simulink model "MMC_AverageModel_20250509"  (R2024b)
settings: Solver=VariableStepAuto  StartTime=0.0  StopTime=0.5  RelTol=1e-3
values from neighbouring files (symbols this model uses):
  Ceq = 3e-3    (= 0.003)    [param_allsim_20250429.m]
  f0 = 50    [param_allsim_20250429.m]
  L_ac = 100e-6    (= 0.0001)    [param_allsim_20250429.m]
  L_arm = 1e-3    (= 0.001)    [param_allsim_20250429.m]
  m_Delta_d = M_Delta*sin(Phi_Delta)    [param_allsim_20250429.m]
  m_Delta_q = -M_Delta*cos(Phi_Delta)    [param_allsim_20250429.m]
  m_Sigma_0 = m_Sigma_0_n    (= 1)    [param_allsim_20250429.m]
  m_Sigma_d = M_Sigma*sin(Phi_Sigma)    [param_allsim_20250429.m]
  m_Sigma_q = -M_Sigma*cos(Phi_Sigma)    [param_allsim_20250429.m]
  R_ac = 1    [param_allsim_20250429.m]
  R_arm = 1e-2    (= 0.01)    [param_allsim_20250429.m]
  VDC = 800    [param_allsim_20250429.m]
undefined symbols (not defined in the file or in its folder): C_SM, Rc
libraries: spsVoltageMeasurementLib x12, spsSeriesRLCBranchLib x12, spsCurrentMeasurementLib x10, spsControlledCurrentSourceLib x6, spsControlledVoltageSourceLib x6, spsabctodq0Lib x6, spsDCVoltageSourceLib x2, spsMeanLib x2, spsdq0toabcLib x2, spsGroundLib x1, spsThreePhaseSeriesRLCBranchLib x1, spspowerguiLib x1
settings Model: Creator=ana  LastModifiedBy=ana

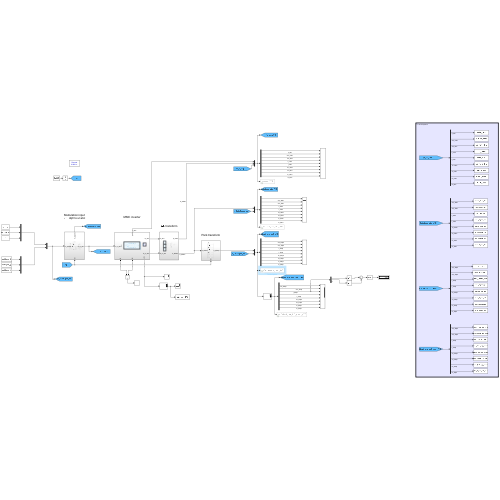
[thumbnail: Simulink's stored preview of the top-level diagram]
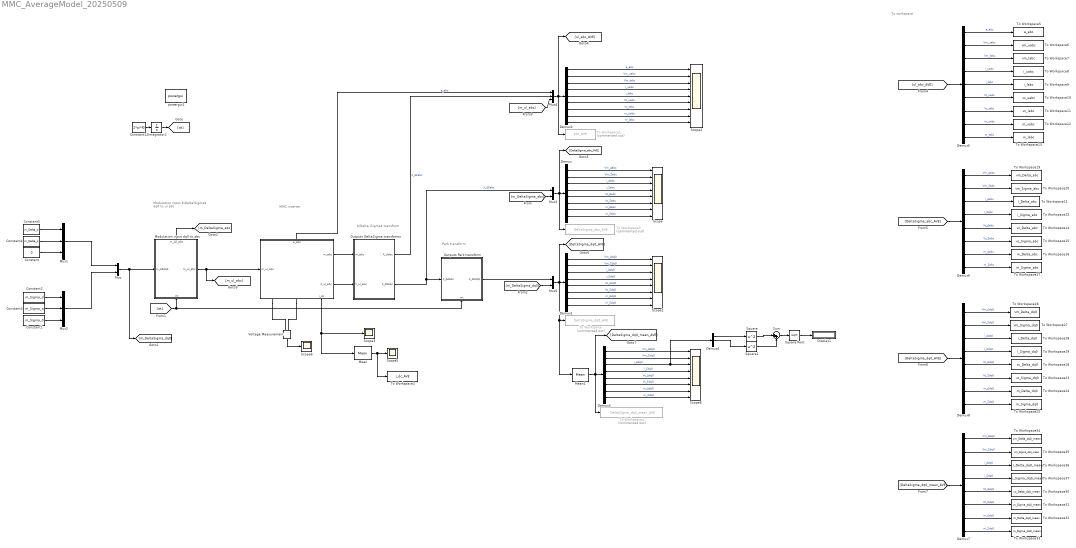
== system MMC_AverageModel_20250509 ==
  note: MMC inverter
  note: $\Delta \Sigma$ transform
  note: Modulation input
      | $\Delta\Sigma$ dq0 to ul abc
  note: Park transform
  note: To workspace
  " " : Subsystem
      settings: PortSchema="{\"entries\":[{\"content\":{\"sides\":[{\"content\":{\"connectorIds\":[\"In1\"]},\"type\":\"ConnectorPlacement.EquallySpacedRectSide\",\"uuid\":\"be96b836-162a-4026-8928-e777e4800056\"},{\"content\":{\"connectorIds\":[\"Out1\",\"Out2\"],\"side\":\"RIGHT\"},\"type\":\"ConnectorPlacement.EquallySpacedRectSide\",\"uuid\":\"77a090ea-e307-4fed-ac75-684872a04d06\"},{\"content\":{\"connectorIds\":[\"Out4\"],\"side\":\"TOP\"},\"type\":\"ConnectorPlacement.EquallySpacedRectSide\",\"uuid\":\"73b87893-2e5b-4437-8911-e3d659e39832\"},{\"content\":{\"connectorIds\":[\"RConn1\",\"RConn2\",\"Out3\"],\"side\":\"BOTTOM\"},\"type\":\"ConnectorPlacement.EquallySpacedRectSide\",\"uuid\":\"828178e9-16e3-463b-9057-d6fa245d9764\"}]},\"type\":\"ConnectorPlacement.EquallySpacedConnector\",\"uuid\":\"6b316bfb-7390-469c-962b-5ea2d8aa7073\"}],\"packageUris\":[\"http://schema.mathworks.com/mf0/Connector/R2020b\"],\"version\":\"1.0\"}"
  Constant : Constant  Value=0
  Constant1 : Constant  Value=m_Sigma_0
  Constant12 : Constant  Value=2*pi*f0
  Constant2 : Constant  Value=m_Sigma_d
  Constant3 : Constant  Value=m_Sigma_q
  Constant4 : Constant  Value=m_Delta_q
  Constant5 : Constant  Value=m_Delta_d
  Demux{,1,3,6..8} (6 alike) : Demux  Outputs=8
  Demux2 : Demux  Outputs=9
  Demux4 : Demux  Outputs=3
  Demux5 : Demux  Outputs=9
  Display1 : Display
  Integrator2 : Integrator
  Mean : spsMeanLib/Mean  Freq=500  Vinit=0  Ts=0
  Mean1 : spsMeanLib/Mean  Freq=500  Vinit=0  Ts=0
  Modulation input dq0 to abc : Subsystem
      settings: PortSchema="{\"entries\":[{\"content\":{\"sides\":[{\"content\":{\"connectorIds\":[\"Out2\"]},\"type\":\"ConnectorPlacement.EquallySpacedRectSide\",\"uuid\":\"c93fa5b4-0f06-4bab-a3ea-c283951bfaa2\"},{\"content\":{\"connectorIds\":[\"In2\"],\"side\":\"RIGHT\"},\"type\":\"ConnectorPlacement.EquallySpacedRectSide\",\"uuid\":\"754fc415-ee26-4c64-88d9-9fe4c190d1ce\"},{\"content\":{\"connectorIds\":[\"Out1\"],\"side\":\"TOP\"},\"type\":\"ConnectorPlacement.EquallySpacedRectSide\",\"uuid\":\"5a2ac060-a673-4c08-b077-b80c57d082e2\"},{\"content\":{\"connectorIds\":[\"In1\"],\"side\":\"BOTTOM\"},\"type\":\"ConnectorPlacement.EquallySpacedRectSide\",\"uuid\":\"ce66d6e2-1782-404f-a52c-1b3df510631d\"}]},\"type\":\"ConnectorPlacement.EquallySpacedConnector\",\"uuid\":\"907f6fc0-1e89-4b6d-bca9-d0cf84d5397d\"}],\"packageUris\":[\"http://schema.mathworks.com/mf0/Connector/R2020b\"],\"version\":\"1.0\"}"
  Mux : Mux  Inputs=2
  Mux1 : Mux  Inputs=3
  Mux2 : Mux  Inputs=3
  Mux3 : Mux  Inputs=2
  Mux4 : Mux  Inputs=3
  Mux5 : Mux  Inputs=2
  Outputs DeltaSigma transforms : Subsystem
      settings: PortSchema="{\"entries\":[{\"content\":{\"sides\":[{\"content\":{\"connectorIds\":[\"Out1\",\"Out2\"]},\"type\":\"ConnectorPlacement.EquallySpacedRectSide\",\"uuid\":\"c93fa5b4-0f06-4bab-a3ea-c283951bfaa2\"},{\"content\":{\"connectorIds\":[\"In1\",\"In2\"],\"side\":\"RIGHT\"},\"type\":\"ConnectorPlacement.EquallySpacedRectSide\",\"uuid\":\"754fc415-ee26-4c64-88d9-9fe4c190d1ce\"},{\"content\":{\"side\":\"TOP\"},\"type\":\"ConnectorPlacement.EquallySpacedRectSide\",\"uuid\":\"5a2ac060-a673-4c08-b077-b80c57d082e2\"},{\"content\":{\"side\":\"BOTTOM\"},\"type\":\"ConnectorPlacement.EquallySpacedRectSide\",\"uuid\":\"ce66d6e2-1782-404f-a52c-1b3df510631d\"}]},\"type\":\"ConnectorPlacement.EquallySpacedConnector\",\"uuid\":\"907f6fc0-1e89-4b6d-bca9-d0cf84d5397d\"}],\"packageUris\":[\"http://schema.mathworks.com/mf0/Connector/R2020b\"],\"version\":\"1.0\"}"
  Outputs Park transform : Subsystem
      settings: PortSchema="{\"entries\":[{\"content\":{\"sides\":[{\"content\":{\"connectorIds\":[\"Out1\"]},\"type\":\"ConnectorPlacement.EquallySpacedRectSide\",\"uuid\":\"c93fa5b4-0f06-4bab-a3ea-c283951bfaa2\"},{\"content\":{\"connectorIds\":[\"In2\"],\"side\":\"RIGHT\"},\"type\":\"ConnectorPlacement.EquallySpacedRectSide\",\"uuid\":\"754fc415-ee26-4c64-88d9-9fe4c190d1ce\"},{\"content\":{\"side\":\"TOP\"},\"type\":\"ConnectorPlacement.EquallySpacedRectSide\",\"uuid\":\"5a2ac060-a673-4c08-b077-b80c57d082e2\"},{\"content\":{\"connectorIds\":[\"In1\"],\"side\":\"BOTTOM\"},\"type\":\"ConnectorPlacement.EquallySpacedRectSide\",\"uuid\":\"ce66d6e2-1782-404f-a52c-1b3df510631d\"}]},\"type\":\"ConnectorPlacement.EquallySpacedConnector\",\"uuid\":\"907f6fc0-1e89-4b6d-bca9-d0cf84d5397d\"}],\"packageUris\":[\"http://schema.mathworks.com/mf0/Connector/R2020b\"],\"version\":\"1.0\"}"
  Scope : Scope  NumInputPorts=8
  Scope1 : Scope  NumInputPorts=8
  Scope2 : Scope  NumInputPorts=9
  Scope3 : Scope
  Scope5 : Scope
  Scope6 : Scope
  Scope8 : Scope  NumInputPorts=8
  Square : Math  Operator=square
  Square Root : Sqrt
  Square1 : Math  Operator=square
  Sum : Sum  Inputs=|++
  To Workspace : ToWorkspace  Commented=on  VariableName=DeltaSigma_dq0_AVE  SaveFormat=Structure With Time  SampleTime=-1
      settings: MaxDataPoints=10*2000
  To Workspace1 : ToWorkspace  Commented=on  VariableName=abc_AVE  SaveFormat=Structure With Time  SampleTime=-1
      settings: MaxDataPoints=10*2000
  To Workspace10 : ToWorkspace  VariableName=vc_uabc  SaveFormat=Structure With Time  SampleTime=-1
      settings: MaxDataPoints=10*200000
  To Workspace11 : ToWorkspace  VariableName=vc_labc  SaveFormat=Structure With Time  SampleTime=-1
      settings: MaxDataPoints=10*200000
  To Workspace12 : ToWorkspace  VariableName=m_uabc  SaveFormat=Structure With Time  SampleTime=-1
      settings: MaxDataPoints=10*200000
  To Workspace13 : ToWorkspace  VariableName=m_labc  SaveFormat=Structure With Time  SampleTime=-1
      settings: MaxDataPoints=10*200000
  To Workspace14 : ToWorkspace  VariableName=vc_Delta_abc  SaveFormat=Structure With Time  SampleTime=-1
      settings: MaxDataPoints=10*200000
  To Workspace15 : ToWorkspace  VariableName=vc_Sigma_abc  SaveFormat=Structure With Time  SampleTime=-1
      settings: MaxDataPoints=10*200000
  To Workspace16 : ToWorkspace  VariableName=m_Delta_abc  SaveFormat=Structure With Time  SampleTime=-1
      settings: MaxDataPoints=10*200000
  To Workspace17 : ToWorkspace  VariableName=m_Sigma_abc  SaveFormat=Structure With Time  SampleTime=-1
      settings: MaxDataPoints=10*200000
  To Workspace18 : ToWorkspace  VariableName=vc_Delta_dq0  SaveFormat=Structure With Time  SampleTime=-1
      settings: MaxDataPoints=10*200000
  To Workspace19 : ToWorkspace  VariableName=vm_Delta_abc  SaveFormat=Structure With Time  SampleTime=-1
      settings: MaxDataPoints=10*200000
  To Workspace2 : ToWorkspace  VariableName=i_dc_AVE  SaveFormat=Structure With Time  SampleTime=-1
      settings: MaxDataPoints=10*2000
  To Workspace20 : ToWorkspace  VariableName=vm_Sigma_abc  SaveFormat=Structure With Time  SampleTime=-1
      settings: MaxDataPoints=10*200000
  To Workspace21 : ToWorkspace  VariableName=i_Delta_abc  SaveFormat=Structure With Time  SampleTime=-1
      settings: MaxDataPoints=10*200000
  To Workspace22 : ToWorkspace  VariableName=i_Sigma_abc  SaveFormat=Structure With Time  SampleTime=-1
      settings: MaxDataPoints=10*200000
  To Workspace23 : ToWorkspace  VariableName=vc_Sigma_dq0  SaveFormat=Structure With Time  SampleTime=-1
      settings: MaxDataPoints=10*200000
  To Workspace24 : ToWorkspace  VariableName=m_Delta_dq0  SaveFormat=Structure With Time  SampleTime=-1
      settings: MaxDataPoints=10*200000
  To Workspace25 : ToWorkspace  VariableName=m_Sigma_dq0  SaveFormat=Structure With Time  SampleTime=-1
      settings: MaxDataPoints=10*200000
  To Workspace26 : ToWorkspace  VariableName=vm_Delta_dq0  SaveFormat=Structure With Time  SampleTime=-1
      settings: MaxDataPoints=10*200000
  To Workspace27 : ToWorkspace  VariableName=vm_Sigma_dq0  SaveFormat=Structure With Time  SampleTime=-1
      settings: MaxDataPoints=10*200000
  To Workspace28 : ToWorkspace  VariableName=i_Delta_dq0  SaveFormat=Structure With Time  SampleTime=-1
      settings: MaxDataPoints=10*200000
  To Workspace29 : ToWorkspace  VariableName=i_Sigma_dq0  SaveFormat=Structure With Time  SampleTime=-1
      settings: MaxDataPoints=10*200000
  To Workspace3 : ToWorkspace  Commented=on  VariableName=DeltaSigma_abc_AVE  SaveFormat=Structure With Time  SampleTime=-1
      settings: MaxDataPoints=10*2000
  To Workspace30 : ToWorkspace  VariableName=vc_Delta_dq0_mean  SaveFormat=Structure With Time  SampleTime=-1
      settings: MaxDataPoints=10*2000
  To Workspace31 : ToWorkspace  VariableName=vc_Sigma_dq0_mean  SaveFormat=Structure With Time  SampleTime=-1
      settings: MaxDataPoints=10*2000
  To Workspace32 : ToWorkspace  VariableName=m_Delta_dq0_mean  SaveFormat=Structure With Time  SampleTime=-1
      settings: MaxDataPoints=10*2000
  To Workspace33 : ToWorkspace  VariableName=m_Sigma_dq0_mean  SaveFormat=Structure With Time  SampleTime=-1
      settings: MaxDataPoints=10*2000
  To Workspace34 : ToWorkspace  VariableName=vm_Delta_dq0_mean  SaveFormat=Structure With Time  SampleTime=-1
      settings: MaxDataPoints=10*2000
  To Workspace35 : ToWorkspace  VariableName=vm_Sigma_dq0_mean  SaveFormat=Structure With Time  SampleTime=-1
      settings: MaxDataPoints=10*2000
  To Workspace36 : ToWorkspace  VariableName=i_Delta_dq0_mean  SaveFormat=Structure With Time  SampleTime=-1
      settings: MaxDataPoints=10*2000
  To Workspace37 : ToWorkspace  VariableName=i_Sigma_dq0_mean  SaveFormat=Structure With Time  SampleTime=-1
      settings: MaxDataPoints=10*2000
  To Workspace4 : ToWorkspace  Commented=on  VariableName=DeltaSigma_dq0_mean_AVE  SaveFormat=Structure With Time  SampleTime=-1
      settings: MaxDataPoints=10*2000
  To Workspace5 : ToWorkspace  VariableName=e_abc  SaveFormat=Structure With Time  SampleTime=-1
      settings: MaxDataPoints=10*200000
  To Workspace6 : ToWorkspace  VariableName=vm_uabc  SaveFormat=Structure With Time  SampleTime=-1
      settings: MaxDataPoints=10*200000
  To Workspace7 : ToWorkspace  VariableName=vm_labc  SaveFormat=Structure With Time  SampleTime=-1
      settings: MaxDataPoints=10*200000
  To Workspace8 : ToWorkspace  VariableName=i_uabc  SaveFormat=Structure With Time  SampleTime=-1
      settings: MaxDataPoints=10*200000
  To Workspace9 : ToWorkspace  VariableName=i_labc  SaveFormat=Structure With Time  SampleTime=-1
      settings: MaxDataPoints=10*200000
  Voltage Measurement : spsVoltageMeasurementLib/Voltage Measurement  PhasorSimulation=off  OutputType=Complex  PSBequivalent=0
  powergui1 : spspowerguiLib/powergui  Priority=1  SimulationMode=Discrete  SampleTime=(1/200)*(1/f0)  frequency=60  Iterations=50  frequencyindice=0  Pbase=100e6  ErrMax=1e-4  UnitsV=V  UnitsW=W  buscounter=0  FunctionMessages=off  echomessages=off  EnableUseOfTLC=off  CurrentSourceSwitches=off  DisableSnubberDevices=off  DisableRonSwitches=off  DisableVfSwitches=off  DisplayEquations=off  AutomaticDiscreteSolvers=off  SolverType=Backward Euler  Interpol=off  ExternalGateDelay=off  methode=off  Ts=0  x0status=blocks  SPID=off  SwTol=0  HookPort=off  NonlinearTolerance=1e-4  nMaxIteration=100  ContinueOnMaxIteration=off  RestoreLinks=warning  ResistiveCurrentMeasurement=off  Frange=[0:2:500]  Ylog=off  Xlog=on  ShowGrid=off  save=off  variable=ZData  structure=0  ZoomFFT=off  StartTime=0.0  cycles=1  DisplayStyle=1  fundamental=60  FreqAxis=off  MaxFrequency=1000  frequencyindicesteady=1  RmsSteady=1  display=off
  wires:
  [wt] -> Outputs Park transform/1(wt), Modulation input dq0 to abc/1(wt)
  Voltage Measurement/1 -> Scope6/1
  Demux2/6 -> Scope2/6  "Vc_uabc"
  Demux3/8 -> Scope8/8  "m_Σdq0"
  Square/1 -> Sum/1
  Demux1/8 -> Scope1/8  "m_Σdq0"
  Mux3/1 -> [DeltaSigma_abc_AVE], To Workspace3/1, Demux/1
  Constant12/1 -> Integrator2/1
  Demux2/8 -> Scope2/8  "m_uabc"
  Demux2/2 -> Scope2/2  "Vm_uabc"
  Integrator2/1 -> [wt]
  Demux/5 -> Scope/5  "Vc_Δabc"
  Square Root/1 -> Display1/1
  Demux/6 -> Scope/6  "Vc_Σabc"
  Demux4/1 -> Square/1
  Sum/1 -> Square Root/1
  Mux/1 -> [m_DeltaSigma_dq0], Modulation input dq0 to abc/2(m_ΔΣdq0)
  Square1/1 -> Sum/2
  " "/3(i_dc) -> Mean/1, Scope3/1
  " "/4(e_abc) -> Mux4/1  "e_abc"
  Demux/3 -> Scope/3  "i_Δabc"
  [m_ul_abc] -> Mux4/3
  Demux3/3 -> Demux4/1, Scope8/3  "i_Δdq0"
  [m_DeltaSigma_abc] -> Mux3/2
  Demux/7 -> Scope/7  "m_Δabc"
  Demux3/7 -> Scope8/7  "m_Δdq0"
  Demux1/5 -> Scope1/5  "Vc_Δdq0"
  Demux3/2 -> Scope8/2  "Vm_Σdq0"
  Constant4/1 -> Mux1/2
  Demux1/3 -> Scope1/3  "i_Δdq0"
  Mux5/1 -> [DeltaSigma_dq0_AVE], Mean1/1, To Workspace/1, Demux1/1
  Demux/4 -> Scope/4  "i_Σabc"
  Demux1/2 -> Scope1/2  "Vm_Σdq0"
  Demux/8 -> Scope/8  "m_Σabc"
  Constant/1 -> Mux1/3
  Demux1/6 -> Scope1/6  "Vc_Σdq0"
  " "/1(m_abc) -> Outputs DeltaSigma transforms/1(m_abc)
  Demux2/7 -> Scope2/7  "Vc_labc"
  Demux2/5 -> Scope2/5  "i_labc"
  Demux4/2 -> Square1/1
  Mean/1 -> To Workspace2/1, Scope5/1
  Demux2/1 -> Scope2/1  "e_abc"
  Demux1/4 -> Scope1/4  "i_Σdq0"
  Demux3/6 -> Scope8/6  "Vc_Σdq0"
  Mux4/1 -> [ul_abc_AVE], Demux2/1, To Workspace1/1
  Constant1/1 -> Mux2/3
  Demux2/9 -> Scope2/9  "m_labc"
  Demux1/7 -> Scope1/7  "m_Δdq0"
  " "/2(X_ul_abc) -> Outputs DeltaSigma transforms/2(X_ul_abc)
  Demux1/1 -> Scope1/1  "Vm_Δdq0"
  Demux3/5 -> Scope8/5  "Vc_Δdq0"
  Modulation input dq0 to abc/1(m_ΔΣ_abc) -> [m_DeltaSigma_abc]
  Demux3/4 -> Scope8/4  "i_Σdq0"
  Outputs Park transform/1("X_ΔΣdq0 ") -> Mux5/1
  Mux2/1 -> Mux/2
  Demux2/4 -> Scope2/4  "i_uabc"
  Outputs DeltaSigma transforms/2(X_ΔΣabc) -> Mux3/1, Outputs Park transform/2("X_ΔΣabc ")  "X_ΔΣabc"
  Outputs DeltaSigma transforms/1(X_ulabc) -> Mux4/2  "X_ΔΣabc"
  Demux/1 -> Scope/1  "Vm_Δabc"
  [m_DeltaSigma_dq0] -> Mux5/2
  Modulation input dq0 to abc/2(m_ul_abc) -> [m_ul_abc], " "/1(m_ul_abc)
  Mux1/1 -> Mux/1
  Demux3/1 -> Scope8/1  "Vm_Δdq0"
  Demux/2 -> Scope/2  "Vm_Σabc"
  Constant5/1 -> Mux1/1
  Constant2/1 -> Mux2/1
  Constant3/1 -> Mux2/2
  Demux2/3 -> Scope2/3  "Vm_labc"
  Mean1/1 -> [DeltaSigma_dq0_mean_AVE], To Workspace4/1, Demux3/1
  Demux5/1 -> To Workspace5/1  "e_abc"
  Demux5/2 -> To Workspace6/1  "Vm_uabc"
  Demux5/3 -> To Workspace7/1  "Vm_labc"
  Demux5/4 -> To Workspace8/1  "i_uabc"
  Demux5/5 -> To Workspace9/1  "i_labc"
  Demux5/6 -> To Workspace10/1  "Vc_uabc"
  Demux5/7 -> To Workspace11/1  "Vc_labc"
  Demux5/8 -> To Workspace12/1  "m_uabc"
  Demux5/9 -> To Workspace13/1  "m_labc"
  [ul_abc_AVE] -> Demux5/1
  [DeltaSigma_abc_AVE] -> Demux6/1
  Demux6/1 -> To Workspace19/1  "Vm_Δabc"
  Demux6/2 -> To Workspace20/1  "Vm_Σabc"
  Demux6/3 -> To Workspace21/1  "i_Δabc"
  Demux6/4 -> To Workspace22/1  "i_Σabc"
  Demux6/5 -> To Workspace14/1  "Vc_Δabc"
  Demux6/6 -> To Workspace15/1  "Vc_Σabc"
  Demux6/7 -> To Workspace16/1  "m_Δabc"
  Demux6/8 -> To Workspace17/1  "m_Σabc"
  Demux7/1 -> To Workspace34/1  "Vm_Δdq0"
  Demux7/2 -> To Workspace35/1  "Vm_Σdq0"
  Demux7/3 -> To Workspace36/1  "i_Δdq0"
  Demux7/4 -> To Workspace37/1  "i_Σdq0"
  Demux7/5 -> To Workspace30/1  "Vc_Δdq0"
  Demux7/6 -> To Workspace31/1  "Vc_Σdq0"
  Demux7/7 -> To Workspace32/1  "m_Δdq0"
  Demux7/8 -> To Workspace33/1  "m_Σdq0"
  Demux8/1 -> To Workspace26/1  "Vm_Δdq0"
  Demux8/2 -> To Workspace27/1  "Vm_Σdq0"
  Demux8/3 -> To Workspace28/1  "i_Δdq0"
  Demux8/4 -> To Workspace29/1  "i_Σdq0"
  Demux8/5 -> To Workspace18/1  "Vc_Δdq0"
  Demux8/6 -> To Workspace23/1  "Vc_Σdq0"
  Demux8/7 -> To Workspace24/1  "m_Δdq0"
  Demux8/8 -> To Workspace25/1  "m_Σdq0"
  [DeltaSigma_dq0_AVE] -> Demux8/1
  [DeltaSigma_dq0_mean_AVE] -> Demux7/1
  connections:
  " "/RConn2 -- Voltage Measurement/LConn2
  " "/RConn1 -- Voltage Measurement/LConn1

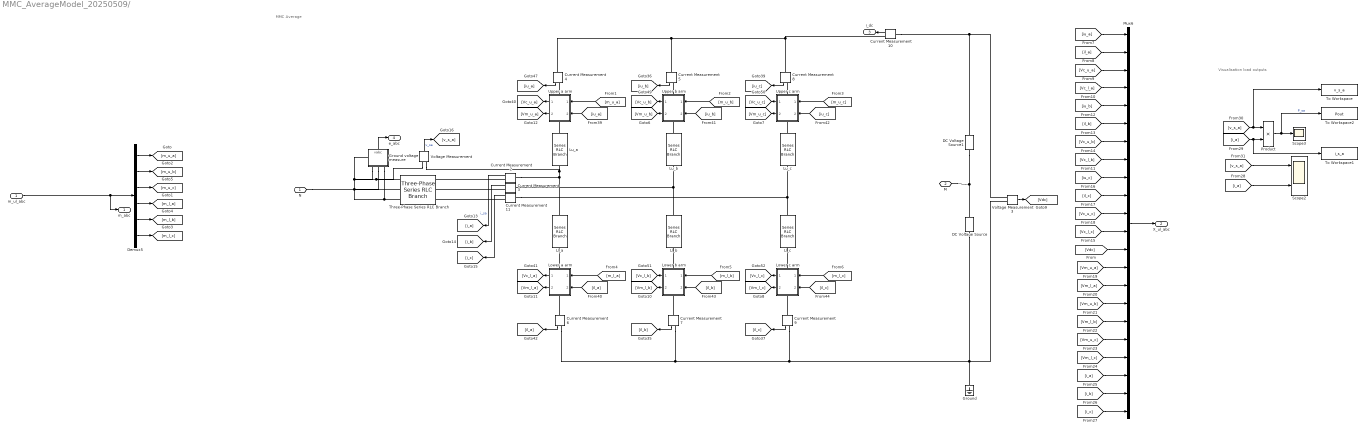
== system MMC_AverageModel_20250509/  ==
  note: MMC Average
  note: Visualisation load outputs
  m_ul_abc : Inport
  Current Measurement{2..11} (10 alike) : spsCurrentMeasurementLib/Current Measurement  PhasorSimulation=off  OutputType=Complex  PSBequivalent=0
  DC Voltage Source : spsDCVoltageSourceLib/DC Voltage Source  Amplitude=VDC/2  Measurements=None
  DC Voltage Source1 : spsDCVoltageSourceLib/DC Voltage Source  Amplitude=VDC/2  Measurements=None
  Demux5 : Demux  Outputs=6
  Ground : spsGroundLib/Ground  LConnTagsString=a
  Ground voltage measure : Subsystem
      settings: PortSchema="{\"entries\":[{\"content\":{\"sides\":[{\"content\":{\"connectorIds\":[\"LConn1\",\"LConn2\",\"LConn3\"]},\"type\":\"ConnectorPlacement.EquallySpacedRectSide\",\"uuid\":\"2d863409-4ac8-4d89-98a2-a138b93b50bd\"},{\"content\":{\"connectorIds\":[\"Out1\"],\"side\":\"RIGHT\"},\"type\":\"ConnectorPlacement.EquallySpacedRectSide\",\"uuid\":\"6b7ceb28-dc80-4bb1-976d-3b9256003f0c\"},{\"content\":{\"connectorIds\":[\"LConn4\"],\"side\":\"TOP\"},\"type\":\"ConnectorPlacement.EquallySpacedRectSide\",\"uuid\":\"b87507a9-fcb6-4c8d-9886-4d479b5c7103\"}]},\"type\":\"ConnectorPlacement.EquallySpacedConnector\",\"uuid\":\"10f317e5-ccdd-49a1-b1ed-441de86b3420\"}],\"packageUris\":[\"http://schema.mathworks.com/mf0/Connector/R2020b\"],\"version\":\"1.0\"}"
  Ll_a : spsSeriesRLCBranchLib/Series RLC Branch  LConnTagsString=__new0  RConnTagsString=__new0  BranchType=RL  Resistance=R_arm  Inductance=L_arm  SetiL0=off  InitialCurrent=0  Capacitance=C_SM  Setx0=off  InitialVoltage=0  Measurements=None
  Ll_b : spsSeriesRLCBranchLib/Series RLC Branch  LConnTagsString=__new0  RConnTagsString=__new0  BranchType=RL  Resistance=R_arm  Inductance=L_arm  SetiL0=off  InitialCurrent=0  Capacitance=C_SM  Setx0=off  InitialVoltage=0  Measurements=None
  Ll_c : spsSeriesRLCBranchLib/Series RLC Branch  LConnTagsString=__new0  RConnTagsString=__new0  BranchType=RL  Resistance=R_arm  Inductance=L_arm  SetiL0=off  InitialCurrent=0  Capacitance=C_SM  Setx0=off  InitialVoltage=0  Measurements=None
  Lower a arm : Subsystem
      settings: PortSchema="{\"entries\":[{\"content\":{\"sides\":[{\"content\":{\"connectorIds\":[\"In1\",\"In2\"]},\"type\":\"ConnectorPlacement.EquallySpacedRectSide\",\"uuid\":\"c73576c4-93d3-495e-8a3c-96adfb3c6bd0\"},{\"content\":{\"connectorIds\":[\"Out1\",\"Out2\"],\"side\":\"RIGHT\"},\"type\":\"ConnectorPlacement.EquallySpacedRectSide\",\"uuid\":\"33fee86c-2024-4810-a753-50b671c6c3a3\"},{\"content\":{\"connectorIds\":[\"LConn1\"],\"side\":\"TOP\"},\"type\":\"ConnectorPlacement.EquallySpacedRectSide\",\"uuid\":\"b34602ad-8a5a-4ef2-987e-97d86aaa7221\"},{\"content\":{\"connectorIds\":[\"RConn1\"],\"side\":\"BOTTOM\"},\"type\":\"ConnectorPlacement.EquallySpacedRectSide\",\"uuid\":\"705e5e9f-0594-4711-b360-8d7f1c1e16a0\"}]},\"type\":\"ConnectorPlacement.EquallySpacedConnector\",\"uuid\":\"05a1ab54-52fb-462c-ba7a-b11a4fb0d277\"}],\"packageUris\":[\"http://schema.mathworks.com/mf0/Connector/R2020b\"],\"version\":\"1.0\"}"
  Lower b arm : Subsystem
      settings: PortSchema="{\"entries\":[{\"content\":{\"sides\":[{\"content\":{\"connectorIds\":[\"In1\",\"In2\"]},\"type\":\"ConnectorPlacement.EquallySpacedRectSide\",\"uuid\":\"c73576c4-93d3-495e-8a3c-96adfb3c6bd0\"},{\"content\":{\"connectorIds\":[\"Out1\",\"Out2\"],\"side\":\"RIGHT\"},\"type\":\"ConnectorPlacement.EquallySpacedRectSide\",\"uuid\":\"33fee86c-2024-4810-a753-50b671c6c3a3\"},{\"content\":{\"connectorIds\":[\"LConn1\"],\"side\":\"TOP\"},\"type\":\"ConnectorPlacement.EquallySpacedRectSide\",\"uuid\":\"b34602ad-8a5a-4ef2-987e-97d86aaa7221\"},{\"content\":{\"connectorIds\":[\"RConn1\"],\"side\":\"BOTTOM\"},\"type\":\"ConnectorPlacement.EquallySpacedRectSide\",\"uuid\":\"705e5e9f-0594-4711-b360-8d7f1c1e16a0\"}]},\"type\":\"ConnectorPlacement.EquallySpacedConnector\",\"uuid\":\"05a1ab54-52fb-462c-ba7a-b11a4fb0d277\"}],\"packageUris\":[\"http://schema.mathworks.com/mf0/Connector/R2020b\"],\"version\":\"1.0\"}"
  Lower c arm : Subsystem
      settings: PortSchema="{\"entries\":[{\"content\":{\"sides\":[{\"content\":{\"connectorIds\":[\"In1\",\"In2\"]},\"type\":\"ConnectorPlacement.EquallySpacedRectSide\",\"uuid\":\"c73576c4-93d3-495e-8a3c-96adfb3c6bd0\"},{\"content\":{\"connectorIds\":[\"Out1\",\"Out2\"],\"side\":\"RIGHT\"},\"type\":\"ConnectorPlacement.EquallySpacedRectSide\",\"uuid\":\"33fee86c-2024-4810-a753-50b671c6c3a3\"},{\"content\":{\"connectorIds\":[\"LConn1\"],\"side\":\"TOP\"},\"type\":\"ConnectorPlacement.EquallySpacedRectSide\",\"uuid\":\"b34602ad-8a5a-4ef2-987e-97d86aaa7221\"},{\"content\":{\"connectorIds\":[\"RConn1\"],\"side\":\"BOTTOM\"},\"type\":\"ConnectorPlacement.EquallySpacedRectSide\",\"uuid\":\"705e5e9f-0594-4711-b360-8d7f1c1e16a0\"}]},\"type\":\"ConnectorPlacement.EquallySpacedConnector\",\"uuid\":\"05a1ab54-52fb-462c-ba7a-b11a4fb0d277\"}],\"packageUris\":[\"http://schema.mathworks.com/mf0/Connector/R2020b\"],\"version\":\"1.0\"}"
  Lu_a : spsSeriesRLCBranchLib/Series RLC Branch  LConnTagsString=__new0  RConnTagsString=__new0  BranchType=RL  Resistance=R_arm  Inductance=L_arm  SetiL0=off  InitialCurrent=0  Capacitance=C_SM  Setx0=off  InitialVoltage=0  Measurements=None
  Lu_b : spsSeriesRLCBranchLib/Series RLC Branch  LConnTagsString=__new0  RConnTagsString=__new0  BranchType=RL  Resistance=R_arm  Inductance=L_arm  SetiL0=off  InitialCurrent=0  Capacitance=C_SM  Setx0=off  InitialVoltage=0  Measurements=None
  Lu_c : spsSeriesRLCBranchLib/Series RLC Branch  LConnTagsString=__new0  RConnTagsString=__new0  BranchType=RL  Resistance=R_arm  Inductance=L_arm  SetiL0=off  InitialCurrent=0  Capacitance=C_SM  Setx0=off  InitialVoltage=0  Measurements=None
  Mux6 : Mux  Inputs=22
  Product : Product
  Scope2 : Scope  NumInputPorts=2
  Scope3 : Scope
  Three-Phase Series RLC Branch : spsThreePhaseSeriesRLCBranchLib/Three-Phase Series RLC Branch  LConnTagsString=A|B|C  RConnTagsString=A|B|C  BranchType=RL  Resistance=R_ac  Inductance=L_ac  Capacitance=1e-6  Measurements=None
  To Workspace : ToWorkspace  VariableName=v_s_a  SaveFormat=Structure With Time  SampleTime=-1
  To Workspace1 : ToWorkspace  VariableName=i_s_a  SaveFormat=Structure With Time  SampleTime=-1
  To Workspace2 : ToWorkspace  VariableName=Pout  SaveFormat=Structure With Time  SampleTime=-1
  Upper a arm : Subsystem
      settings: PortSchema="{\"entries\":[{\"content\":{\"sides\":[{\"content\":{\"connectorIds\":[\"In1\",\"In2\"]},\"type\":\"ConnectorPlacement.EquallySpacedRectSide\",\"uuid\":\"c73576c4-93d3-495e-8a3c-96adfb3c6bd0\"},{\"content\":{\"connectorIds\":[\"Out1\",\"Out2\"],\"side\":\"RIGHT\"},\"type\":\"ConnectorPlacement.EquallySpacedRectSide\",\"uuid\":\"33fee86c-2024-4810-a753-50b671c6c3a3\"},{\"content\":{\"connectorIds\":[\"LConn1\"],\"side\":\"TOP\"},\"type\":\"ConnectorPlacement.EquallySpacedRectSide\",\"uuid\":\"b34602ad-8a5a-4ef2-987e-97d86aaa7221\"},{\"content\":{\"connectorIds\":[\"RConn1\"],\"side\":\"BOTTOM\"},\"type\":\"ConnectorPlacement.EquallySpacedRectSide\",\"uuid\":\"705e5e9f-0594-4711-b360-8d7f1c1e16a0\"}]},\"type\":\"ConnectorPlacement.EquallySpacedConnector\",\"uuid\":\"05a1ab54-52fb-462c-ba7a-b11a4fb0d277\"}],\"packageUris\":[\"http://schema.mathworks.com/mf0/Connector/R2020b\"],\"version\":\"1.0\"}"
  Upper b arm : Subsystem
      settings: PortSchema="{\"entries\":[{\"content\":{\"sides\":[{\"content\":{\"connectorIds\":[\"In1\",\"In2\"]},\"type\":\"ConnectorPlacement.EquallySpacedRectSide\",\"uuid\":\"c73576c4-93d3-495e-8a3c-96adfb3c6bd0\"},{\"content\":{\"connectorIds\":[\"Out1\",\"Out2\"],\"side\":\"RIGHT\"},\"type\":\"ConnectorPlacement.EquallySpacedRectSide\",\"uuid\":\"33fee86c-2024-4810-a753-50b671c6c3a3\"},{\"content\":{\"connectorIds\":[\"LConn1\"],\"side\":\"TOP\"},\"type\":\"ConnectorPlacement.EquallySpacedRectSide\",\"uuid\":\"b34602ad-8a5a-4ef2-987e-97d86aaa7221\"},{\"content\":{\"connectorIds\":[\"RConn1\"],\"side\":\"BOTTOM\"},\"type\":\"ConnectorPlacement.EquallySpacedRectSide\",\"uuid\":\"705e5e9f-0594-4711-b360-8d7f1c1e16a0\"}]},\"type\":\"ConnectorPlacement.EquallySpacedConnector\",\"uuid\":\"05a1ab54-52fb-462c-ba7a-b11a4fb0d277\"}],\"packageUris\":[\"http://schema.mathworks.com/mf0/Connector/R2020b\"],\"version\":\"1.0\"}"
  Upper c arm : Subsystem
      settings: PortSchema="{\"entries\":[{\"content\":{\"sides\":[{\"content\":{\"connectorIds\":[\"In1\",\"In2\"]},\"type\":\"ConnectorPlacement.EquallySpacedRectSide\",\"uuid\":\"c73576c4-93d3-495e-8a3c-96adfb3c6bd0\"},{\"content\":{\"connectorIds\":[\"Out1\",\"Out2\"],\"side\":\"RIGHT\"},\"type\":\"ConnectorPlacement.EquallySpacedRectSide\",\"uuid\":\"33fee86c-2024-4810-a753-50b671c6c3a3\"},{\"content\":{\"connectorIds\":[\"LConn1\"],\"side\":\"TOP\"},\"type\":\"ConnectorPlacement.EquallySpacedRectSide\",\"uuid\":\"b34602ad-8a5a-4ef2-987e-97d86aaa7221\"},{\"content\":{\"connectorIds\":[\"RConn1\"],\"side\":\"BOTTOM\"},\"type\":\"ConnectorPlacement.EquallySpacedRectSide\",\"uuid\":\"705e5e9f-0594-4711-b360-8d7f1c1e16a0\"}]},\"type\":\"ConnectorPlacement.EquallySpacedConnector\",\"uuid\":\"05a1ab54-52fb-462c-ba7a-b11a4fb0d277\"}],\"packageUris\":[\"http://schema.mathworks.com/mf0/Connector/R2020b\"],\"version\":\"1.0\"}"
  Voltage Measurement : spsVoltageMeasurementLib/Voltage Measurement  PhasorSimulation=off  OutputType=Complex  PSBequivalent=0
  Voltage Measurement3 : spsVoltageMeasurementLib/Voltage Measurement  PhasorSimulation=off  OutputType=Complex  PSBequivalent=0
  N : PMIOPort  Side=Right
  M : PMIOPort  Port=2  Side=Right
  m_abc : Outport
  X_ul_abc : Outport  Port=2
  i_dc : Outport  Port=3
  e_abc : Outport  Port=4
  wires:
  Demux5/1 -> [m_u_a]
  [iu_a] -> Mux6/1
  [il_a] -> Mux6/2
  [Vc_u_a] -> Mux6/3
  [Vc_l_a] -> Mux6/4
  [iu_b] -> Mux6/5
  [il_b] -> Mux6/6
  [Vc_u_b] -> Mux6/7
  [Vc_l_b] -> Mux6/8
  [iu_c] -> Mux6/9
  [il_c] -> Mux6/10
  [Vc_u_c] -> Mux6/11
  [Vc_l_c] -> Mux6/12
  Mux6/1 -> X_ul_abc/1
  [Vdc] -> Mux6/13
  Lower b arm/2(Vm_l_b) -> [Vm_l_b]
  Lower c arm/1(Vc_l_c) -> [Vc_l_c]
  Upper b arm/2(Vm_u_b) -> [Vm_u_b]
  Upper c arm/1(Vc_u_c) -> [Vc_u_c]
  Current Measurement8/1 -> [iu_c]
  [il_b] -> Lower b arm/2(I_l_b)
  Lower a arm/1(Vc_l_a) -> [Vc_l_a]
  Current Measurement6/1 -> [il_a]
  [iu_b] -> Upper b arm/2(I_u_b)
  Lower a arm/2(Vm_l_a) -> [Vm_l_a]
  [m_l_b] -> Lower b arm/1(m_l_b)
  [m_u_c] -> Upper c arm/1(m_u_c)
  [m_u_b] -> Upper b arm/1(m_u_b)
  [il_a] -> Lower a arm/2(I_l_a)
  Voltage Measurement3/1 -> [Vdc]
  [iu_a] -> Upper a arm/2(I_u_a)
  [m_u_a] -> Upper a arm/1(m_u_a)
  Current Measurement4/1 -> [iu_a]
  [il_c] -> Lower c arm/2(I_l_c)
  [iu_c] -> Upper c arm/2(I_u_c)
  Current Measurement7/1 -> [il_b]
  Current Measurement5/1 -> [iu_b]
  [m_l_c] -> Lower c arm/1(m_l_c)
  Current Measurement9/1 -> [il_c]
  Upper a arm/2(Vm_u_a) -> [Vm_u_a]
  Upper c arm/2(Vm_u_c) -> [Vm_u_c]
  Upper b arm/1(Vc_u_b) -> [Vc_u_b]
  Lower c arm/2(Vm_l_c) -> [Vm_l_c]
  Upper a arm/1(Vc_u_a) -> [Vc_u_a]
  Lower b arm/1(Vc_l_b) -> [Vc_l_b]
  [m_l_a] -> Lower a arm/1(m_l_a)
  Current Measurement10/1 -> i_dc/1
  [Vm_u_a] -> Mux6/14
  [Vm_l_a] -> Mux6/15
  [Vm_u_b] -> Mux6/16
  [Vm_l_b] -> Mux6/17
  [Vm_u_c] -> Mux6/18
  [Vm_l_c] -> Mux6/19
  Demux5/2 -> [m_u_b]
  Demux5/3 -> [m_u_c]
  Demux5/5 -> [m_l_b]
  Demux5/6 -> [m_l_c]
  Demux5/4 -> [m_l_a]
  Ground voltage measure/1(vabc) -> e_abc/1
  m_ul_abc/1 -> Demux5/1, m_abc/1
  Current Measurement2/1 -> [i_a]  "i_sa"
  Current Measurement3/1 -> [i_b]
  Current Measurement11/1 -> [i_c]
  [i_a] -> Mux6/20
  [i_b] -> Mux6/21
  [i_c] -> Mux6/22
  Product/1 -> To Workspace2/1, Scope3/1  "P_sa"
  Voltage Measurement/1 -> [v_s_a]  "v_sa"
  [i_a] -> Scope2/2
  [i_a] -> Product/2, To Workspace1/1
  [v_s_a] -> To Workspace/1, Product/1
  [v_s_a] -> Scope2/1
  connections:
  Ll_c/LConn1 -- Current Measurement11/LConn1 -- Lu_c/RConn1
  Ll_b/LConn1 -- Current Measurement3/LConn1 -- Lu_b/RConn1
  Current Measurement8/LConn1 -- Current Measurement10/RConn1 -- Current Measurement5/LConn1 -- Current Measurement4/LConn1
  Lu_a/RConn1 -- Ll_a/LConn1 -- Current Measurement2/LConn1 -- Voltage Measurement/LConn1
  Current Measurement7/LConn1 -- Lower b arm/RConn1
  Lu_b/LConn1 -- Upper b arm/RConn1
  Lu_a/LConn1 -- Upper a arm/RConn1
  Current Measurement6/LConn1 -- Lower a arm/RConn1
  Lu_c/LConn1 -- Upper c arm/RConn1
  Upper a arm/LConn1 -- Current Measurement4/RConn1
  Ll_b/RConn1 -- Lower b arm/LConn1
  Current Measurement9/LConn1 -- Lower c arm/RConn1
  Upper c arm/LConn1 -- Current Measurement8/RConn1
  Ll_c/RConn1 -- Lower c arm/LConn1
  Upper b arm/LConn1 -- Current Measurement5/RConn1
  Lower a arm/LConn1 -- Ll_a/RConn1
  DC Voltage Source1/LConn1 -- M/RConn1 -- DC Voltage Source/RConn1
  Current Measurement10/LConn1 -- DC Voltage Source1/RConn1 -- Voltage Measurement3/LConn1
  Ground voltage measure/LConn3 -- Ground voltage measure/LConn4 -- Ground voltage measure/LConn1 -- Voltage Measurement/LConn2 -- Three-Phase Series RLC Branch/RConn1 -- Ground voltage measure/LConn2 -- Three-Phase Series RLC Branch/RConn2 -- N/RConn1 -- Three-Phase Series RLC Branch/RConn3
  Voltage Measurement3/LConn2 -- Ground/LConn1 -- Current Measurement9/RConn1 -- Current Measurement7/RConn1 -- Current Measurement6/RConn1 -- DC Voltage Source/LConn1
  Current Measurement2/RConn1 -- Three-Phase Series RLC Branch/LConn1
  Current Measurement3/RConn1 -- Three-Phase Series RLC Branch/LConn2
  Current Measurement11/RConn1 -- Three-Phase Series RLC Branch/LConn3

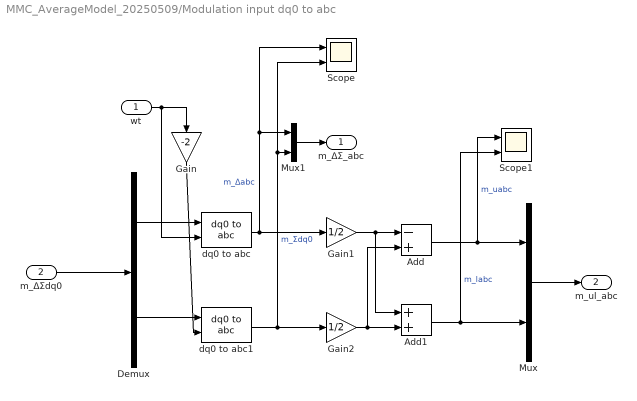
== system MMC_AverageModel_20250509/Modulation input dq0 to abc ==
  wt : Inport
  m_ΔΣdq0 : Inport  Port=2
  Add : Sum  Inputs=-+
  Add1 : Sum
  Demux : Demux  Outputs=2
  Gain : Gain  Gain=-2
  Gain1 : Gain  Gain=1/2
  Gain2 : Gain  Gain=1/2
  Mux : Mux  Inputs=2
  Mux1 : Mux  Inputs=2
  Scope : Scope  NumInputPorts=2
  Scope1 : Scope  NumInputPorts=2
  dq0 to abc : spsdq0toabcLib/dq0 to abc  Alignment=Aligned with phase A axis
  dq0 to abc1 : spsdq0toabcLib/dq0 to abc  Alignment=Aligned with phase A axis
  m_ΔΣ_abc : Outport
  m_ul_abc : Outport  Port=2
  wires:
  m_ΔΣdq0/1 -> Demux/1
  wt/1 -> dq0 to abc/2, Gain/1
  Mux/1 -> m_ul_abc/1
  Demux/1 -> dq0 to abc/1
  Demux/2 -> dq0 to abc1/1
  Gain/1 -> dq0 to abc1/2
  dq0 to abc/1 -> Scope/1, Mux1/1, Gain1/1  "m_Δabc"
  dq0 to abc1/1 -> Scope/2, Mux1/2, Gain2/1  "m_Σdq0"
  Gain2/1 -> Add/2, Add1/2
  Gain1/1 -> Add1/1, Add/1
  Add/1 -> Scope1/1, Mux/1  "m_uabc"
  Add1/1 -> Scope1/2, Mux/2  "m_labc"
  Mux1/1 -> m_ΔΣ_abc/1

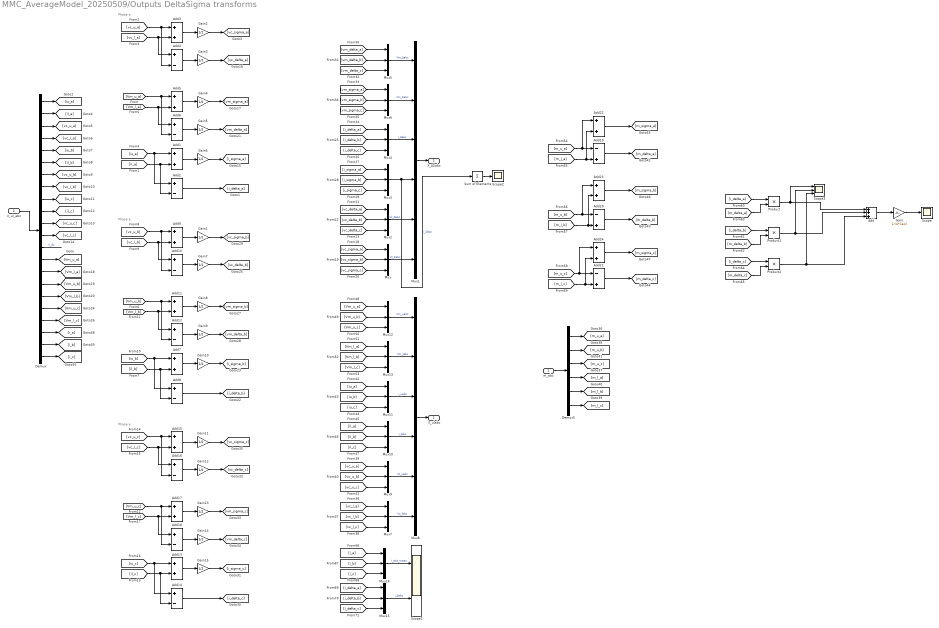
== system MMC_AverageModel_20250509/Outputs DeltaSigma transforms ==
  note: Phase a
  note: Phase a
  note: Phase a
  m_abc : Inport
  X_ul_abc : Inport  Port=2
  Add : Sum  Inputs=+++
  Add{1,3,5,7,9,11,13,15,17,22..24} (12 alike) : Sum
  Add{2,4,6,8,10,12,14,16,18} (9 alike) : Sum  Inputs=+-
  Add19 : Sum  Inputs=-+
  Add20 : Sum  Inputs=-+
  Add21 : Sum  Inputs=-+
  Demux : Demux  Outputs=22
  Demux5 : Demux  Outputs=6
  Gain : Gain  Gain=1/(4*Ceq)
  Gain{1..15} (15 alike) : Gain  Gain=1/2
  Mux{,2..7,9..15} (14 alike) : Mux  Inputs=3
  Mux1 : Mux  Inputs=6
  Mux8 : Mux  Inputs=6
  Product : Product
  Product1 : Product
  Product2 : Product
  Scope : Scope
  Scope1 : Scope  NumInputPorts=2
  Scope2 : Scope
  Scope3 : Scope  NumInputPorts=3
  Sum of Elements : Sum  Inputs=+
  X_ulabc : Outport
  X_ΔΣabc : Outport  Port=2
  wires:
  X_ul_abc/1 -> Demux/1
  Demux/1 -> [iu_a]
  Demux/2 -> [il_a]
  Demux/3 -> [vc_u_a]
  Demux/4 -> [vc_l_a]
  Demux/5 -> [iu_b]
  Demux/6 -> [il_b]
  Demux/7 -> [vc_u_b]
  Demux/8 -> [vc_l_b]
  Demux/9 -> [iu_c]
  Demux/10 -> [il_c]
  Demux/11 -> [vc_u_c]
  Demux/12 -> [vc_l_c]
  [iu_a] -> Add2/1, Add1/1
  [vc_l_a] -> Add4/1, Add3/2
  [vc_u_a] -> Add4/2, Add3/1
  Gain2/1 -> [vc_sigma_a]
  Add1/1 -> Gain6/1
  Add3/1 -> Gain2/1
  [il_a] -> Add2/2, Add1/2
  Demux/14 -> [Vm_u_a]
  Demux/15 -> [Vm_l_a]
  Demux/16 -> [Vm_u_b]
  Demux/17 -> [Vm_l_b]
  Demux/18 -> [Vm_u_c]
  Demux/19 -> [Vm_l_c]
  Add4/1 -> Gain3/1
  Gain3/1 -> [vc_delta_a]
  Gain5/1 -> [vm_delta_a]
  Add6/1 -> Gain5/1
  Add5/1 -> Gain4/1
  [Vm_l_a] -> Add6/1, Add5/2
  Gain4/1 -> [vm_sigma_a]
  [Vm_u_a] -> Add6/2, Add5/1
  Add2/1 -> [i_delta_a]
  Gain6/1 -> [i_sigma_a]
  Gain8/1 -> [vm_sigma_b]
  Add11/1 -> Gain8/1
  Gain7/1 -> [vc_delta_b]
  Add10/1 -> Gain7/1
  [Vm_u_b] -> Add12/2, Add11/1
  Add9/1 -> Gain1/1
  [il_b] -> Add8/2, Add7/2
  Add7/1 -> Gain10/1
  Gain9/1 -> [vm_delta_b]
  [iu_b] -> Add8/1, Add7/1
  [vc_u_b] -> Add10/2, Add9/1
  Gain1/1 -> [vc_sigma_b]
  Add12/1 -> Gain9/1
  Add8/1 -> [i_delta_b]
  Gain10/1 -> [i_sigma_b]
  [Vm_l_b] -> Add12/1, Add11/2
  [vc_l_b] -> Add10/1, Add9/2
  Gain13/1 -> [vm_sigma_c]
  Add17/1 -> Gain13/1
  Gain12/1 -> [vc_delta_c]
  Add16/1 -> Gain12/1
  [Vm_u_c] -> Add18/2, Add17/1
  Add15/1 -> Gain11/1
  [il_c] -> Add14/2, Add13/2
  Add13/1 -> Gain15/1
  Gain14/1 -> [vm_delta_c]
  [iu_c] -> Add14/1, Add13/1
  [vc_u_c] -> Add16/2, Add15/1
  Gain11/1 -> [vc_sigma_c]
  Add18/1 -> Gain14/1
  Add14/1 -> [i_delta_c]
  Gain15/1 -> [i_sigma_c]
  [Vm_l_c] -> Add18/1, Add17/2
  [vc_l_c] -> Add16/1, Add15/2
  [vc_sigma_a] -> Mux/1
  [vc_sigma_b] -> Mux/2
  [vc_sigma_c] -> Mux/3
  [vc_delta_a] -> Mux2/1
  [vc_delta_b] -> Mux2/2
  [vc_delta_c] -> Mux2/3
  Mux2/1 -> Mux1/5  "Vc_Δabc"
  Mux/1 -> Mux1/6  "Vc_Σabc"
  Mux3/1 -> Sum of Elements/1, Mux1/4  "i_Σabc"
  [i_sigma_c] -> Mux3/3
  [i_sigma_b] -> Mux3/2
  [i_sigma_a] -> Mux3/1
  Mux4/1 -> Mux1/3  "i_Δabc"
  [i_delta_a] -> Mux4/1
  [i_delta_b] -> Mux4/2
  [i_delta_c] -> Mux4/3
  [vm_delta_b] -> Mux5/2
  [vm_delta_c] -> Mux5/3
  Mux5/1 -> Mux1/1  "Vm_Δabc"
  [vm_delta_a] -> Mux5/1
  [vm_sigma_a] -> Mux6/1
  [vm_sigma_c] -> Mux6/3
  [vm_sigma_b] -> Mux6/2
  Mux6/1 -> Mux1/2  "Vm_Σabc"
  Mux1/1 -> X_ΔΣabc/1
  [Vm_l_b] -> Mux13/2
  Mux9/1 -> Mux8/5  "Vc_uabc"
  [Vm_u_a] -> Mux12/1
  [vc_l_c] -> Mux7/3
  Mux10/1 -> Mux8/4  "i_labc"
  [il_b] -> Mux10/2
  [vc_u_c] -> Mux9/3
  [iu_b] -> Mux11/2
  [il_a] -> Mux10/1
  [Vm_l_a] -> Mux13/1
  [vc_l_a] -> Mux7/1
  [vc_l_b] -> Mux7/2
  [Vm_l_c] -> Mux13/3
  [iu_c] -> Mux11/3
  [vc_u_b] -> Mux9/2
  Mux11/1 -> Mux8/3  "i_uabc"
  [Vm_u_c] -> Mux12/3
  Mux13/1 -> Mux8/2  "Vm_labc"
  [il_c] -> Mux10/3
  [Vm_u_b] -> Mux12/2
  Mux7/1 -> Mux8/6  "Vc_labc"
  [iu_a] -> Mux11/1
  Mux8/1 -> X_ulabc/1
  Mux12/1 -> Mux8/1  "Vm_uabc"
  [vc_u_a] -> Mux9/1
  Demux/13 -> ?  "V_dc"
  m_abc/1 -> Demux5/1
  Demux5/4 -> [m_l_a]
  Demux5/6 -> [m_l_c]
  Demux5/5 -> [m_l_b]
  Demux5/3 -> [m_u_c]
  Demux5/2 -> [m_u_b]
  Demux5/1 -> [m_u_a]
  [m_l_a] -> Add22/2, Add19/2
  [m_u_a] -> Add22/1, Add19/1
  Add19/1 -> [m_delta_a]
  [m_u_b] -> Add23/1, Add20/1
  Add20/1 -> [m_delta_b]
  [m_l_b] -> Add23/2, Add20/2
  [m_u_c] -> Add24/1, Add21/1
  Add21/1 -> [m_delta_c]
  [m_l_c] -> Add24/2, Add21/2
  Add22/1 -> [m_sigma_a]
  Add23/1 -> [m_sigma_b]
  Add24/1 -> [m_sigma_c]
  [i_delta_a] -> Product/1
  [m_delta_a] -> Product/2
  [i_delta_b] -> Product1/1
  [m_delta_b] -> Product1/2
  [i_delta_c] -> Product2/1
  [m_delta_c] -> Product2/2
  Product/1 -> Scope3/1, Add/1
  Product1/1 -> Scope3/2, Add/2
  Product2/1 -> Scope3/3, Add/3
  Add/1 -> Gain/1
  Gain/1 -> Scope/1
  Sum of Elements/1 -> Scope2/1
  Demux/20 -> [i_a]
  Demux/21 -> [i_b]
  Demux/22 -> [i_c]
  [i_delta_c] -> Mux15/3
  [i_delta_b] -> Mux15/2
  [i_delta_a] -> Mux15/1
  [i_a] -> Mux14/1
  [i_b] -> Mux14/2
  [i_c] -> Mux14/3
  Mux14/1 -> Scope1/1  "I_abc_meas"
  Mux15/1 -> Scope1/2  "i_Δabc"

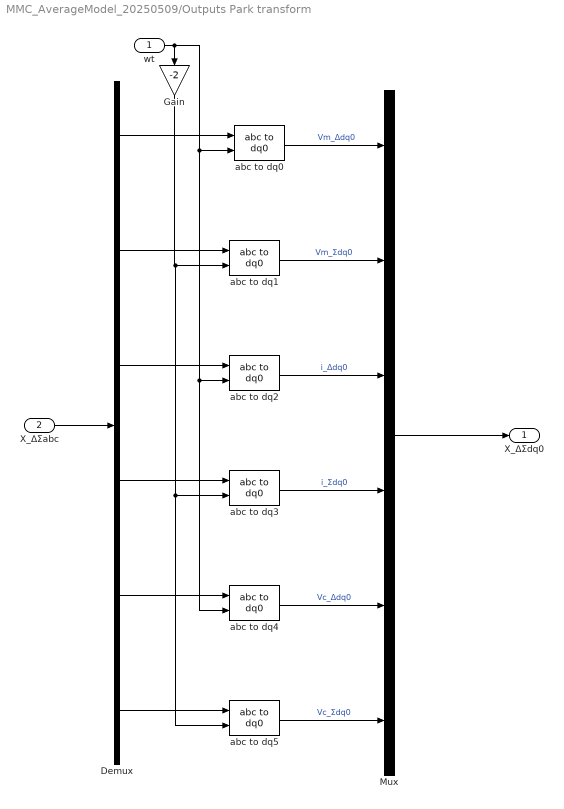
== system MMC_AverageModel_20250509/Outputs Park transform ==
  wt : Inport
  "X_ΔΣabc " : Inport  Port=2
  Demux : Demux  Outputs=6
  Gain : Gain  Gain=-2
  Mux : Mux  Inputs=6
  abc to dq{0..5} (6 alike) : spsabctodq0Lib/abc to dq0  Alignment=Aligned with phase A axis
  "X_ΔΣdq0 " : Outport
  wires:
  "X_ΔΣabc "/1 -> Demux/1
  Demux/1 -> abc to dq0/1
  wt/1 -> Gain/1, abc to dq4/2, abc to dq2/2, abc to dq0/2
  abc to dq0/1 -> Mux/1  "Vm_Δdq0"
  abc to dq1/1 -> Mux/2  "Vm_Σdq0"
  abc to dq2/1 -> Mux/3  "i_Δdq0"
  abc to dq3/1 -> Mux/4  "i_Σdq0"
  abc to dq4/1 -> Mux/5  "Vc_Δdq0"
  abc to dq5/1 -> Mux/6  "Vc_Σdq0"
  Gain/1 -> abc to dq1/2, abc to dq5/2, abc to dq3/2
  Demux/2 -> abc to dq1/1
  Demux/3 -> abc to dq2/1
  Demux/4 -> abc to dq3/1
  Demux/5 -> abc to dq4/1
  Demux/6 -> abc to dq5/1
  Mux/1 -> "X_ΔΣdq0 "/1

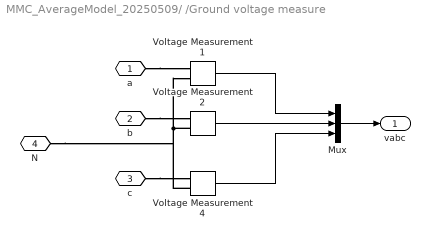
== system MMC_AverageModel_20250509/ /Ground voltage measure ==
  Mux : Mux  Inputs=3
  Voltage Measurement1 : spsVoltageMeasurementLib/Voltage Measurement  PhasorSimulation=off  OutputType=Complex  PSBequivalent=0
  Voltage Measurement2 : spsVoltageMeasurementLib/Voltage Measurement  PhasorSimulation=off  OutputType=Complex  PSBequivalent=0
  Voltage Measurement4 : spsVoltageMeasurementLib/Voltage Measurement  PhasorSimulation=off  OutputType=Complex  PSBequivalent=0
  a : PMIOPort  Side=Left
  b : PMIOPort  Port=2  Side=Left
  c : PMIOPort  Port=3  Side=Left
  N : PMIOPort  Port=4  Side=Left
  vabc : Outport
  wires:
  Voltage Measurement4/1 -> Mux/3
  Voltage Measurement2/1 -> Mux/2
  Mux/1 -> vabc/1
  Voltage Measurement1/1 -> Mux/1
  connections:
  Voltage Measurement2/LConn2 -- Voltage Measurement4/LConn2 -- N/RConn1 -- Voltage Measurement1/LConn2
  a/RConn1 -- Voltage Measurement1/LConn1
  b/RConn1 -- Voltage Measurement2/LConn1
  c/RConn1 -- Voltage Measurement4/LConn1

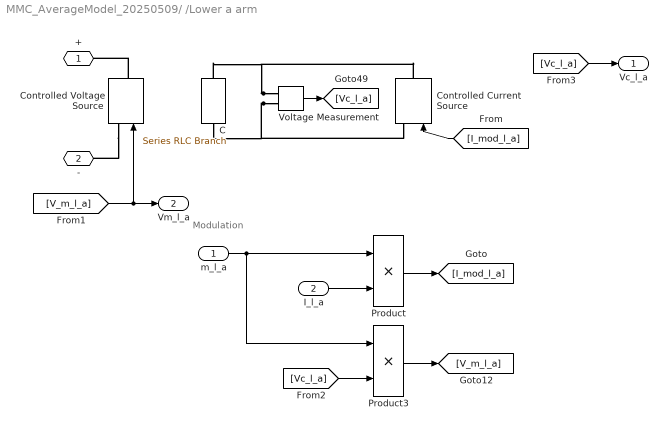
== system MMC_AverageModel_20250509/ /Lower a arm ==
  note: Modulation
  m_l_a : Inport
  I_l_a : Inport  Port=2
  C : spsSeriesRLCBranchLib/Series RLC Branch  LConnTagsString=__new0  RConnTagsString=__new0  BranchType=C  Resistance=Rc  Inductance=100e-6  SetiL0=on  InitialCurrent=0  Capacitance=Ceq  Setx0=on  InitialVoltage=VDC  Measurements=None
  Controlled Current Source : spsControlledCurrentSourceLib/Controlled Current Source  Initialize=on  Source_Type=AC  Amplitude=0  Phase=0  Frequency=0  Measurements=None
  Controlled Voltage Source : spsControlledVoltageSourceLib/Controlled Voltage Source  Initialize=on  Source_Type=AC  Amplitude=0  Phase=0  Frequency=0  Measurements=None
  Product : Product
  Product3 : Product
  Voltage Measurement : spsVoltageMeasurementLib/Voltage Measurement  PhasorSimulation=off  OutputType=Complex  PSBequivalent=0
  + : PMIOPort  Side=Left
  - : PMIOPort  Port=2  Side=Right
  Vc_l_a : Outport
  Vm_l_a : Outport  Port=2
  wires:
  Voltage Measurement/1 -> [Vc_l_a]
  Product/1 -> [I_mod_l_a]
  I_l_a/1 -> Product/2
  [Vc_l_a] -> Product3/2
  Product3/1 -> [V_m_l_a]
  m_l_a/1 -> Product3/1, Product/1
  [V_m_l_a] -> Vm_l_a/1, Controlled Voltage Source/1
  [I_mod_l_a] -> Controlled Current Source/1
  [Vc_l_a] -> Vc_l_a/1
  connections:
  Voltage Measurement/LConn1 -- C/LConn1 -- Controlled Current Source/RConn1
  Voltage Measurement/LConn2 -- C/RConn1 -- Controlled Current Source/LConn1
  Controlled Voltage Source/RConn1 -- +/RConn1
  Controlled Voltage Source/LConn1 -- -/RConn1

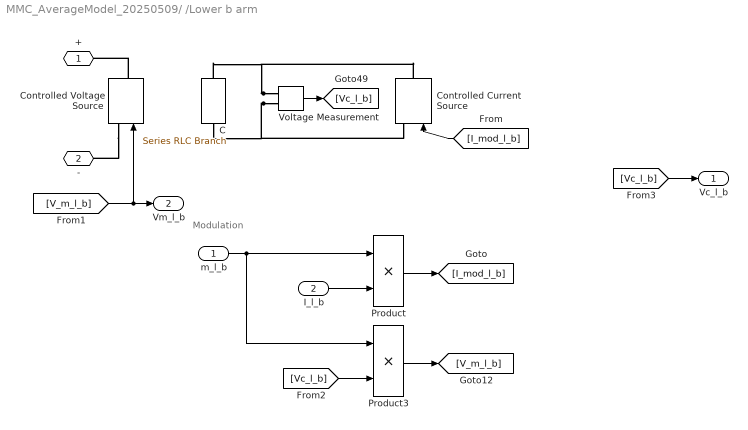
== system MMC_AverageModel_20250509/ /Lower b arm ==
  note: Modulation
  m_l_b : Inport
  I_l_b : Inport  Port=2
  C : spsSeriesRLCBranchLib/Series RLC Branch  LConnTagsString=__new0  RConnTagsString=__new0  BranchType=C  Resistance=Rc  Inductance=100e-6  SetiL0=on  InitialCurrent=0  Capacitance=Ceq  Setx0=on  InitialVoltage=VDC  Measurements=None
  Controlled Current Source : spsControlledCurrentSourceLib/Controlled Current Source  Initialize=on  Source_Type=AC  Amplitude=0  Phase=0  Frequency=0  Measurements=None
  Controlled Voltage Source : spsControlledVoltageSourceLib/Controlled Voltage Source  Initialize=on  Source_Type=AC  Amplitude=0  Phase=0  Frequency=0  Measurements=None
  Product : Product
  Product3 : Product
  Voltage Measurement : spsVoltageMeasurementLib/Voltage Measurement  PhasorSimulation=off  OutputType=Complex  PSBequivalent=0
  + : PMIOPort  Side=Left
  - : PMIOPort  Port=2  Side=Right
  Vc_l_b : Outport
  Vm_l_b : Outport  Port=2
  wires:
  Voltage Measurement/1 -> [Vc_l_b]
  Product/1 -> [I_mod_l_b]
  I_l_b/1 -> Product/2
  [Vc_l_b] -> Product3/2
  Product3/1 -> [V_m_l_b]
  m_l_b/1 -> Product3/1, Product/1
  [V_m_l_b] -> Vm_l_b/1, Controlled Voltage Source/1
  [I_mod_l_b] -> Controlled Current Source/1
  [Vc_l_b] -> Vc_l_b/1
  connections:
  Voltage Measurement/LConn1 -- C/LConn1 -- Controlled Current Source/RConn1
  Voltage Measurement/LConn2 -- C/RConn1 -- Controlled Current Source/LConn1
  Controlled Voltage Source/RConn1 -- +/RConn1
  Controlled Voltage Source/LConn1 -- -/RConn1

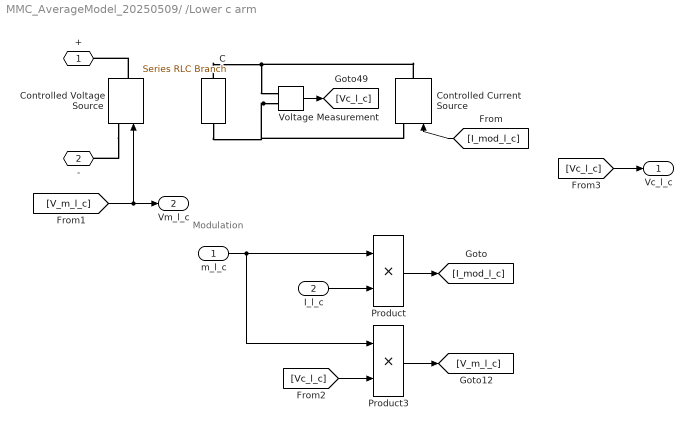
== system MMC_AverageModel_20250509/ /Lower c arm ==
  note: Modulation
  m_l_c : Inport
  I_l_c : Inport  Port=2
  C : spsSeriesRLCBranchLib/Series RLC Branch  LConnTagsString=__new0  RConnTagsString=__new0  BranchType=C  Resistance=Rc  Inductance=100e-6  SetiL0=on  InitialCurrent=0  Capacitance=Ceq  Setx0=on  InitialVoltage=VDC  Measurements=None
  Controlled Current Source : spsControlledCurrentSourceLib/Controlled Current Source  Initialize=on  Source_Type=AC  Amplitude=0  Phase=0  Frequency=0  Measurements=None
  Controlled Voltage Source : spsControlledVoltageSourceLib/Controlled Voltage Source  Initialize=on  Source_Type=AC  Amplitude=0  Phase=0  Frequency=0  Measurements=None
  Product : Product
  Product3 : Product
  Voltage Measurement : spsVoltageMeasurementLib/Voltage Measurement  PhasorSimulation=off  OutputType=Complex  PSBequivalent=0
  + : PMIOPort  Side=Left
  - : PMIOPort  Port=2  Side=Right
  Vc_l_c : Outport
  Vm_l_c : Outport  Port=2
  wires:
  Voltage Measurement/1 -> [Vc_l_c]
  Product/1 -> [I_mod_l_c]
  I_l_c/1 -> Product/2
  [Vc_l_c] -> Product3/2
  Product3/1 -> [V_m_l_c]
  m_l_c/1 -> Product3/1, Product/1
  [V_m_l_c] -> Controlled Voltage Source/1, Vm_l_c/1
  [I_mod_l_c] -> Controlled Current Source/1
  [Vc_l_c] -> Vc_l_c/1
  connections:
  C/LConn1 -- Voltage Measurement/LConn1 -- Controlled Current Source/RConn1
  Voltage Measurement/LConn2 -- C/RConn1 -- Controlled Current Source/LConn1
  Controlled Voltage Source/RConn1 -- +/RConn1
  Controlled Voltage Source/LConn1 -- -/RConn1

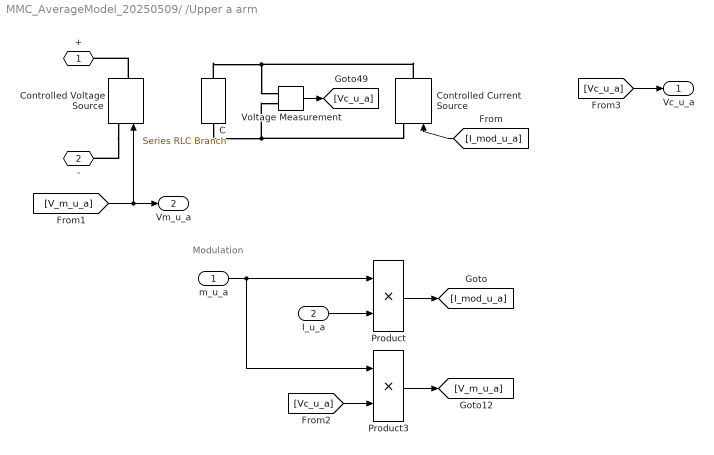
== system MMC_AverageModel_20250509/ /Upper a arm ==
  note: Modulation
  m_u_a : Inport
  I_u_a : Inport  Port=2
  C : spsSeriesRLCBranchLib/Series RLC Branch  LConnTagsString=__new0  RConnTagsString=__new0  BranchType=C  Resistance=Rc  Inductance=100e-6  SetiL0=on  InitialCurrent=0  Capacitance=Ceq  Setx0=on  InitialVoltage=VDC  Measurements=None
  Controlled Current Source : spsControlledCurrentSourceLib/Controlled Current Source  Initialize=on  Source_Type=AC  Amplitude=0  Phase=0  Frequency=0  Measurements=None
  Controlled Voltage Source : spsControlledVoltageSourceLib/Controlled Voltage Source  Initialize=on  Source_Type=AC  Amplitude=0  Phase=0  Frequency=0  Measurements=None
  Product : Product
  Product3 : Product
  Voltage Measurement : spsVoltageMeasurementLib/Voltage Measurement  PhasorSimulation=off  OutputType=Complex  PSBequivalent=0
  + : PMIOPort  Side=Left
  - : PMIOPort  Port=2  Side=Right
  Vc_u_a : Outport
  Vm_u_a : Outport  Port=2
  wires:
  Voltage Measurement/1 -> [Vc_u_a]
  Product/1 -> [I_mod_u_a]
  I_u_a/1 -> Product/2
  [Vc_u_a] -> Product3/2
  Product3/1 -> [V_m_u_a]
  m_u_a/1 -> Product3/1, Product/1
  [V_m_u_a] -> Controlled Voltage Source/1, Vm_u_a/1
  [I_mod_u_a] -> Controlled Current Source/1
  [Vc_u_a] -> Vc_u_a/1
  connections:
  Controlled Current Source/RConn1 -- C/LConn1 -- Voltage Measurement/LConn1
  Controlled Current Source/LConn1 -- C/RConn1 -- Voltage Measurement/LConn2
  Controlled Voltage Source/RConn1 -- +/RConn1
  Controlled Voltage Source/LConn1 -- -/RConn1

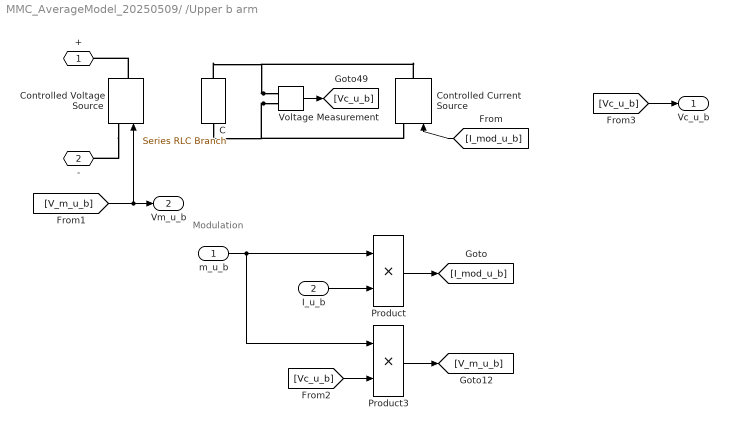
== system MMC_AverageModel_20250509/ /Upper b arm ==
  note: Modulation
  m_u_b : Inport
  I_u_b : Inport  Port=2
  C : spsSeriesRLCBranchLib/Series RLC Branch  LConnTagsString=__new0  RConnTagsString=__new0  BranchType=C  Resistance=Rc  Inductance=100e-6  SetiL0=on  InitialCurrent=0  Capacitance=Ceq  Setx0=on  InitialVoltage=VDC  Measurements=None
  Controlled Current Source : spsControlledCurrentSourceLib/Controlled Current Source  Initialize=on  Source_Type=AC  Amplitude=0  Phase=0  Frequency=0  Measurements=None
  Controlled Voltage Source : spsControlledVoltageSourceLib/Controlled Voltage Source  Initialize=on  Source_Type=AC  Amplitude=0  Phase=0  Frequency=0  Measurements=None
  Product : Product
  Product3 : Product
  Voltage Measurement : spsVoltageMeasurementLib/Voltage Measurement  PhasorSimulation=off  OutputType=Complex  PSBequivalent=0
  + : PMIOPort  Side=Left
  - : PMIOPort  Port=2  Side=Right
  Vc_u_b : Outport
  Vm_u_b : Outport  Port=2
  wires:
  Voltage Measurement/1 -> [Vc_u_b]
  Product/1 -> [I_mod_u_b]
  I_u_b/1 -> Product/2
  [Vc_u_b] -> Product3/2
  Product3/1 -> [V_m_u_b]
  m_u_b/1 -> Product3/1, Product/1
  [V_m_u_b] -> Vm_u_b/1, Controlled Voltage Source/1
  [I_mod_u_b] -> Controlled Current Source/1
  [Vc_u_b] -> Vc_u_b/1
  connections:
  Voltage Measurement/LConn1 -- C/LConn1 -- Controlled Current Source/RConn1
  Voltage Measurement/LConn2 -- C/RConn1 -- Controlled Current Source/LConn1
  Controlled Voltage Source/RConn1 -- +/RConn1
  Controlled Voltage Source/LConn1 -- -/RConn1

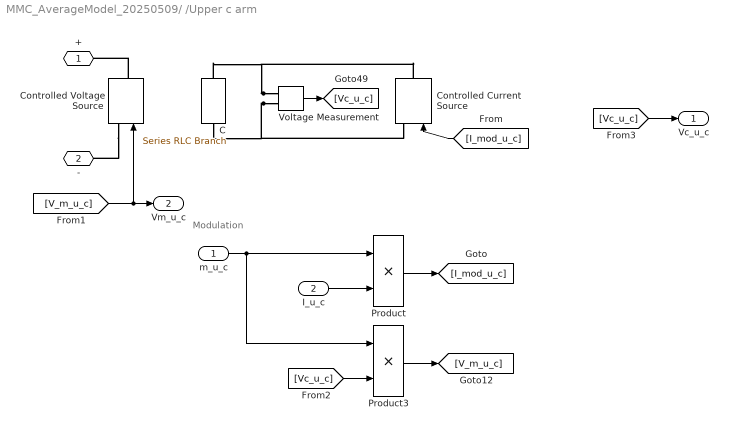
== system MMC_AverageModel_20250509/ /Upper c arm ==
  note: Modulation
  m_u_c : Inport
  I_u_c : Inport  Port=2
  C : spsSeriesRLCBranchLib/Series RLC Branch  LConnTagsString=__new0  RConnTagsString=__new0  BranchType=C  Resistance=Rc  Inductance=100e-6  SetiL0=on  InitialCurrent=0  Capacitance=Ceq  Setx0=on  InitialVoltage=VDC  Measurements=None
  Controlled Current Source : spsControlledCurrentSourceLib/Controlled Current Source  Initialize=on  Source_Type=AC  Amplitude=0  Phase=0  Frequency=0  Measurements=None
  Controlled Voltage Source : spsControlledVoltageSourceLib/Controlled Voltage Source  Initialize=on  Source_Type=AC  Amplitude=0  Phase=0  Frequency=0  Measurements=None
  Product : Product
  Product3 : Product
  Voltage Measurement : spsVoltageMeasurementLib/Voltage Measurement  PhasorSimulation=off  OutputType=Complex  PSBequivalent=0
  + : PMIOPort  Side=Left
  - : PMIOPort  Port=2  Side=Right
  Vc_u_c : Outport
  Vm_u_c : Outport  Port=2
  wires:
  Voltage Measurement/1 -> [Vc_u_c]
  Product/1 -> [I_mod_u_c]
  I_u_c/1 -> Product/2
  [Vc_u_c] -> Product3/2
  Product3/1 -> [V_m_u_c]
  m_u_c/1 -> Product3/1, Product/1
  [V_m_u_c] -> Vm_u_c/1, Controlled Voltage Source/1
  [I_mod_u_c] -> Controlled Current Source/1
  [Vc_u_c] -> Vc_u_c/1
  connections:
  Voltage Measurement/LConn1 -- C/LConn1 -- Controlled Current Source/RConn1
  Voltage Measurement/LConn2 -- C/RConn1 -- Controlled Current Source/LConn1
  Controlled Voltage Source/RConn1 -- +/RConn1
  Controlled Voltage Source/LConn1 -- -/RConn1
